simulink model "simulacion1"  (R2015a)
settings: Solver=ode3  StartTime=0.0  StopTime=10  FixedStep=1  RelTol=1e-3
settings Model: Creator=Jesus  LastModifiedBy=Jesus

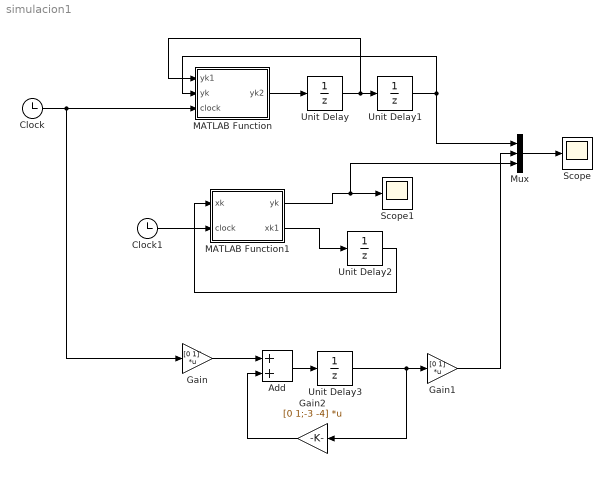
== system simulacion1 ==
  Add : Sum
  Clock : Clock
  Clock1 : Clock
  Gain : Gain  Gain=[0 1]'  Multiplication=Matrix(K*u)
  Gain1 : Gain  Gain=[0 1]  Multiplication=Matrix(K*u)
  Gain2 : Gain  Gain=[0 1;-3 -4]  Multiplication=Matrix(K*u)
  MATLAB Function : MATLAB Function  TreatAsAtomicUnit=on
  MATLAB Function1 : MATLAB Function  TreatAsAtomicUnit=on
  Mux : Mux  Inputs=3
  Scope : Scope
      settings: YMin=-800  YMax=400
  Scope1 : Scope
  Unit Delay : UnitDelay  InitialCondition=1  SampleTime=-1
  Unit Delay1 : UnitDelay  InitialCondition=-1  SampleTime=-1
  Unit Delay2 : UnitDelay  InitialCondition=[1 -1]  SampleTime=-1
  Unit Delay3 : UnitDelay  InitialCondition=[1 -1]  SampleTime=-1
  wires:
  Unit Delay/1 -> MATLAB Function/1(yk1), Unit Delay1/1
  Unit Delay1/1 -> MATLAB Function/2(yk), Mux/1
  MATLAB Function/1(yk2) -> Unit Delay/1
  MATLAB Function1/2(xk1) -> Unit Delay2/1
  Unit Delay2/1 -> MATLAB Function1/1(xk)
  Mux/1 -> Scope/1
  Gain/1 -> Add/1
  Add/1 -> Unit Delay3/1
  Unit Delay3/1 -> Gain2/1, Gain1/1
  Gain2/1 -> Add/2
  Gain1/1 -> Mux/2
  MATLAB Function1/1(yk) -> Mux/3, Scope1/1
  Clock/1 -> MATLAB Function/3(clock), Gain/1
  Clock1/1 -> MATLAB Function1/2(clock)

== matlab function simulacion1/MATLAB Function1 ==
  data: yk output; xk input; xk1 output; clock input
function [yk,xk1] = fcn(xk,clock)
%#codegen
uk=clock;
A=[0 1;-3 -4];
B=[0 1]';
C=[0 1];
xk1= A*xk + B*uk;
yk=C*xk;

== matlab function simulacion1/MATLAB Function ==
  data: yk1 input; yk2 output; yk input; clock input
function yk2 = fcn(yk1,yk,clock)
%#codegen
uk1=clock+1;
yk2=-4*yk1-3*yk+uk1;
